simulink model "ADC_RunningAvg_Test"  (R2022b)
settings: Solver=VariableStepAuto  StartTime=0.0  StopTime=170  RelTol=1e-3
libraries: dspstat3 x1, simulink x1, SignalEditorBlockLib x1
settings Model: Creator=LinF  LastModifiedBy=LinF

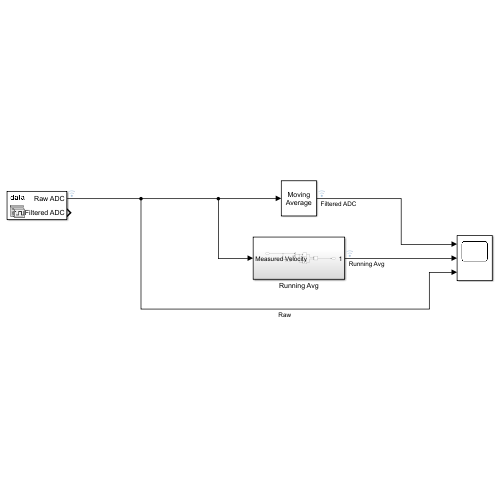
[thumbnail: Simulink's stored preview of the top-level diagram]
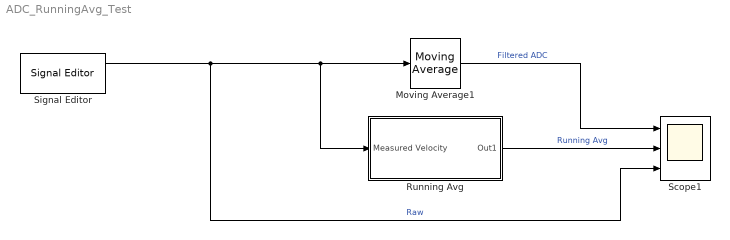
== system ADC_RunningAvg_Test ==
  Moving Average1 : dspstat3/Moving Average  Method=Exponential weighting  ForgettingFactorPort=off  SpecifyWindowLength=on  WindowLength=4  OverlapLength=3  AllowArbitraryInputLength=off  ForgettingFactor=0.8  SimulateUsing=Code generation
  Running Avg : Subsystem
  Scope1 : Scope  NumInputPorts=3
  Signal Editor : SignalEditorBlockLib/Signal Editor  FileName=ADC_Noise.mat  ActiveScenario=data  ActiveSignal=Raw ADC  IsBus=off  OutputBusObjectStr=Bus: BusObject  SampleTime=0.005  Interpolate=off  ZeroCross=off  OutputAfterFinalValue=Setting to zero  Unit=inherit  PreserveSignalName=on
  wires:
  Moving Average1/1 -> Scope1/1  "Filtered ADC"
  Running Avg/1(Out1) -> Scope1/2  "Running Avg"
  Signal Editor/1 -> Scope1/3, Running Avg/1(Measured Velocity), Moving Average1/1  "Raw"

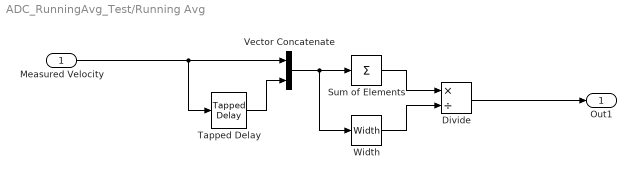
== system ADC_RunningAvg_Test/Running Avg ==
  Measured Velocity : Inport
  Divide : Product  Inputs=*/
  Sum of Elements : Sum  Inputs=+
  Tapped Delay : simulink/Discrete/Tapped Delay  vinit=0  samptime=-1  NumDelays=5  DelayOrder=Oldest  includeCurrent=off
  Vector Concatenate : Concatenate
  Width : Width
  Out1 : Outport
  wires:
  Divide/1 -> Out1/1
  Vector Concatenate/1 -> Width/1, Sum of Elements/1
  Measured Velocity/1 -> Vector Concatenate/1, Tapped Delay/1
  Width/1 -> Divide/2
  Tapped Delay/1 -> Vector Concatenate/2
  Sum of Elements/1 -> Divide/1
